simulink model "lyskawaLab5_si"  (R2023b)
settings: Solver=VariableStepAuto  StartTime=0.0  StopTime=10.0  MaxStep=0.01  RelTol=1e-3
values from neighbouring files (symbols this model uses):
  du = 1    [lyskawaLab5.m]
  ksi = ksi_s(i)    [lyskawaLab5.m]
  t0 = 0    [lyskawaLab5.m]
  u0 = 0    [lyskawaLab5.m]
  w = w_s(i)    [lyskawaLab5.m]
  x0 = 0    [lyskawaLab5.m]
  xDot0 = 0    [lyskawaLab5.m]
settings Model: Creator=aleklyskawa  LastModifiedBy=aleklyskawa

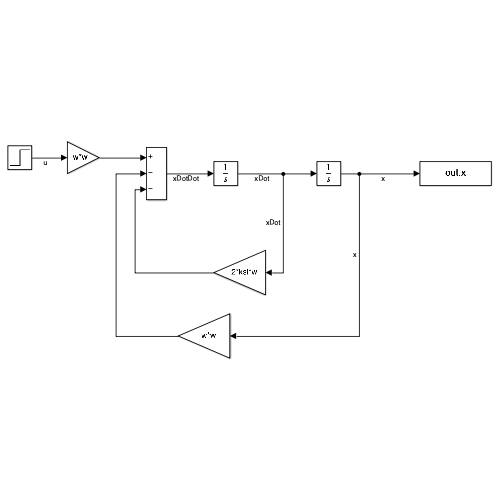
[thumbnail: Simulink's stored preview of the top-level diagram]
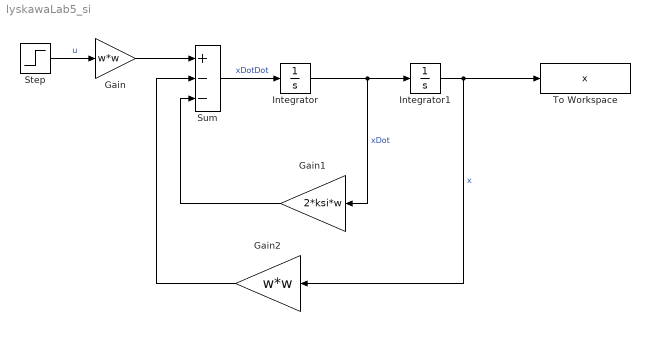
== system lyskawaLab5_si ==
  Gain : Gain  Gain=w*w
  Gain1 : Gain  Gain=2*ksi*w
  Gain2 : Gain  Gain=w*w
  Integrator : Integrator  InitialCondition=xDot0
  Integrator1 : Integrator  InitialCondition=x0
  Step : Step  Time=t0  Before=u0  After=u0 + du  SampleTime=0
  Sum : Sum  Inputs=+--
  To Workspace : ToWorkspace  VariableName=x  SampleTime=-1
  wires:
  Step/1 -> Gain/1  "u"
  Gain/1 -> Sum/1
  Sum/1 -> Integrator/1  "xDotDot"
  Integrator/1 -> Gain1/1, Integrator1/1  "xDot"
  Gain1/1 -> Sum/3
  Integrator1/1 -> Gain2/1, To Workspace/1  "x"
  Gain2/1 -> Sum/2
